simulink model "cp_aero_machineside"  (R2023b)
settings: Solver=VariableStepAuto  StartTime=0.0  StopTime=100  RelTol=1e-3
undefined symbols (not defined in the file): c_drt, C_p_opt, H_gen, H_WTR, k_drt, K_pitch, ki, kp, L_d, L_q, lambda_opt, omega_WTR_0, omega_WTR_min, omega_WTR_n, omega_WTR_sl0, pitch_max, pitch_min, poles, psi_pm, R_a, R_WTR, rate_max, rate_min, T_pitch, T_servo, v_w_n, wind_array_step
libraries: spsdq0toabcLib x1
settings Model: Creator=Martin Pedersen  LastModifiedBy=s183702

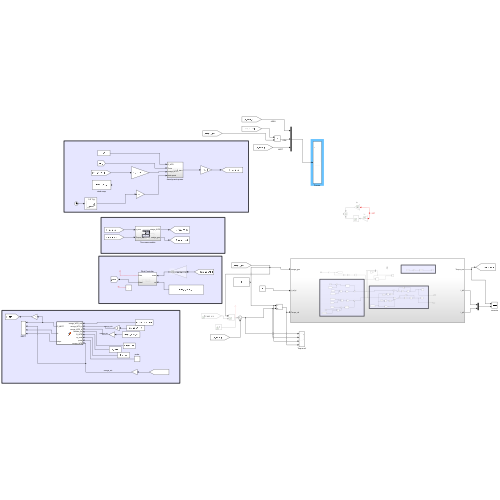
[thumbnail: Simulink's stored preview of the top-level diagram]
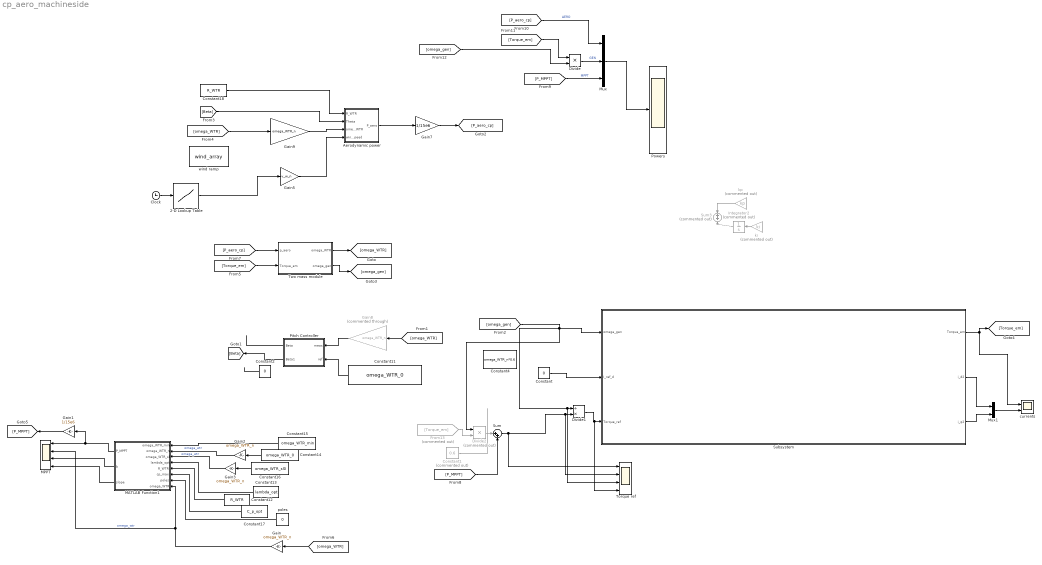
== system cp_aero_machineside ==
  2-D Lookup Table : Lookup_n-D  NumberOfTableDimensions=1  BreakpointsForDimension1=wind_array_step(1,:)  BreakpointsForDimension2=[1:3]  IndexSearchMethod=Linear search  Table=wind_array_step(2,:)  InterpMethod=Nearest  InternalRulePriority=Speed  RndMeth=Simplest
  Aerodynamic power : Subsystem
  Clock : Clock
  Constant : Constant  Value=0
  Constant1 : Constant  Commented=on  Value=0.6
  Constant11 : Constant  Value=omega_WTR_0
  Constant12 : Constant  Value=R_WTR
  Constant13 : Constant  Value=lambda_opt
  Constant14 : Constant  Value=omega_WTR_0
  Constant15 : Constant  Value=omega_WTR_min
  Constant16 : Constant  Value=omega_WTR_sl0
  Constant17 : Constant  Value=C_p_opt
  Constant18 : Constant  Value=R_WTR
  Constant2 : Constant  Value=0
  Constant4 : Constant  Value=omega_WTR_n*0.6
  Divide : Product  Inputs=**
  Divide1 : Product  Inputs=/*
  Divide2 : Product  Commented=on  Inputs=**
  From13 : From  Commented=on  GotoTag=Torque_em
  Gain{,2..3,9} (4 alike) : Gain  Gain=omega_WTR_n
  Gain1 : Gain  Gain=1/15e6
  Gain5 : Gain  Gain=v_w_n
  Gain7 : Gain  Gain=1/15e6
  Gain8 : Gain  Commented=through  Gain=omega_WTR_n
  Integrator2 : Integrator  Commented=on
  MATLAB Function1 : MATLAB Function  TreatAsAtomicUnit=on
  MPPT : Scope  NumInputPorts=4
  Mux : Mux  Inputs=3
  Mux1 : Mux  Inputs=2
  Pitch Controller : Subsystem
  Powers : Scope
  Subsystem : Subsystem
  Sum : Sum  Inputs=|++
  Sum3 : Sum  Commented=on  Inputs=+|+
  Torque ref : Scope  NumInputPorts=4
  Two mass module : Subsystem
  currents : Scope  NumInputPorts=2
  ki : Gain  Commented=on  Gain=ki
  kp : Gain  Commented=on  Gain=kp
  poles : Constant  Value=0
  wind ramp : FromWorkspace  VariableName=wind_array
  wires:
  Gain7/1 -> [P_aero_cp]
  [omega_WTR] -> Gain9/1
  Constant18/1 -> Aerodynamic power/1(R_WTR)
  [Beta] -> Aerodynamic power/2(Theta)
  Gain9/1 -> Aerodynamic power/3(omega_WTR)
  Gain5/1 -> Aerodynamic power/4(wind speed)
  Aerodynamic power/1(P_aero) -> Gain7/1
  MATLAB Function1/3(slope) -> MPPT/4
  MATLAB Function1/2(b) -> MPPT/3
  MATLAB Function1/1(P_MPPT) -> Gain1/1, MPPT/1
  Constant16/1 -> Gain3/1
  Constant17/1 -> MATLAB Function1/6(cp_max)
  Constant13/1 -> MATLAB Function1/4(lambda_opt)
  poles/1 -> MATLAB Function1/7(poles)
  Gain/1 -> MATLAB Function1/8(omega_WTR), MPPT/2  "omega_wtr"
  Constant12/1 -> MATLAB Function1/5(R_WTR)
  Constant14/1 -> Gain2/1
  Constant15/1 -> MATLAB Function1/1(omega_WTR_min)
  Two mass module/1(omega_WTR) -> [omega_WTR]
  [omega_WTR] -> Gain8/1
  Gain8/1 -> Pitch Controller/1(meas)
  Constant11/1 -> Pitch Controller/2(ref)
  kp/1 -> Sum3/1
  ? -> ki/1, kp/1
  ki/1 -> Integrator2/1
  Integrator2/1 -> Sum3/2
  Two mass module/2(omega_gen) -> [omega_gen]
  Subsystem/1(Torque_em) -> [Torque_em], currents/1
  [Torque_em] -> Two mass module/2(Torque_em)
  [omega_WTR] -> Gain/1
  [P_aero_cp] -> Two mass module/1(p_aero)
  Constant/1 -> Subsystem/2(I_ref_d)
  [P_MPPT] -> Mux/3  "MPPT"
  [P_aero_cp] -> Mux/1  "AERO"
  Divide/1 -> Mux/2  "GEN"
  [Torque_em] -> Divide/1
  Gain1/1 -> [P_MPPT]
  Mux1/1 -> currents/2
  Subsystem/2(i_d2) -> Mux1/1
  Subsystem/3(i_q2) -> Mux1/2
  Mux/1 -> Powers/1
  Pitch Controller/1(Beta) -> ?
  2-D Lookup Table/1 -> Gain5/1
  [omega_gen] -> Divide/2
  Constant2/1 -> ?
  Divide1/1 -> Torque ref/4, Subsystem/3(Torque_ref)
  Divide2/1 -> ?
  [P_MPPT] -> Sum/2
  Sum/1 -> Torque ref/2, Divide1/2, Torque ref/1
  Constant1/1 -> Sum/1
  From13/1 -> Divide2/2
  Gain2/1 -> MATLAB Function1/2(omega_WTR_n)  "omega_wtr"
  Gain3/1 -> MATLAB Function1/3(omega_WTR_sl)  "omega_wtr"
  [omega_gen] -> Torque ref/3, Divide1/1, Divide2/1, Subsystem/1(omega_gen)
  Pitch Controller/2(Beta1) -> [Beta]
  Clock/1 -> 2-D Lookup Table/1

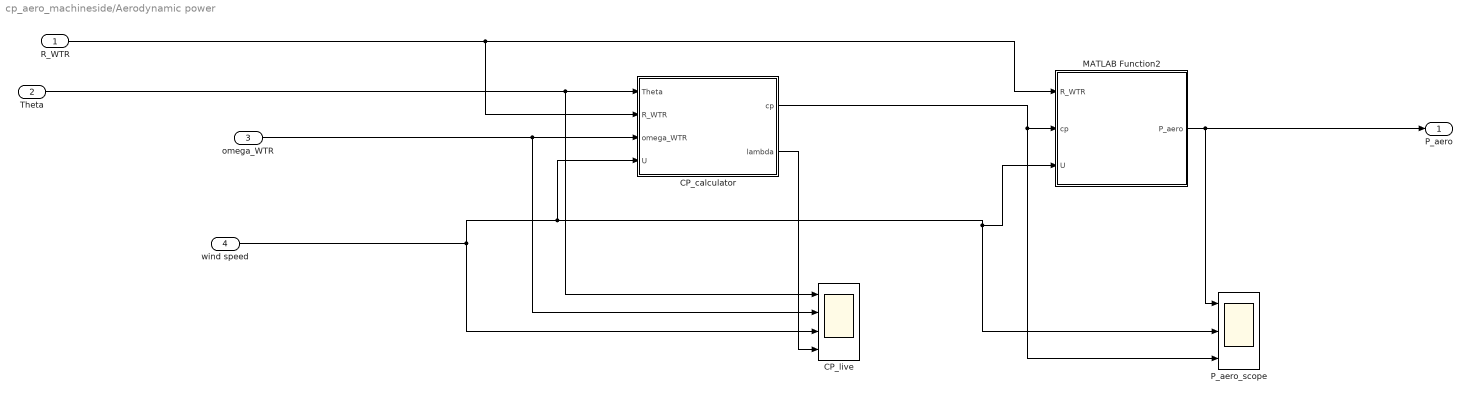
== system cp_aero_machineside/Aerodynamic power ==
  R_WTR : Inport
  Theta : Inport  Port=2
  omega_WTR : Inport  Port=3
  wind speed : Inport  Port=4
  CP_calculator : MATLAB Function  TreatAsAtomicUnit=on
  CP_live : Scope  NumInputPorts=4
  MATLAB Function2 : MATLAB Function  TreatAsAtomicUnit=on
  P_aero_scope : Scope  NumInputPorts=3
  P_aero : Outport
  wires:
  R_WTR/1 -> CP_calculator/2(R_WTR), MATLAB Function2/1(R_WTR)
  CP_calculator/1(cp) -> P_aero_scope/3, MATLAB Function2/2(cp)
  wind speed/1 -> P_aero_scope/2, MATLAB Function2/3(U), CP_calculator/4(U), CP_live/3
  Theta/1 -> CP_live/1, CP_calculator/1(Theta)
  omega_WTR/1 -> CP_calculator/3(omega_WTR), CP_live/2
  MATLAB Function2/1(P_aero) -> P_aero/1, P_aero_scope/1
  CP_calculator/2(lambda) -> CP_live/4

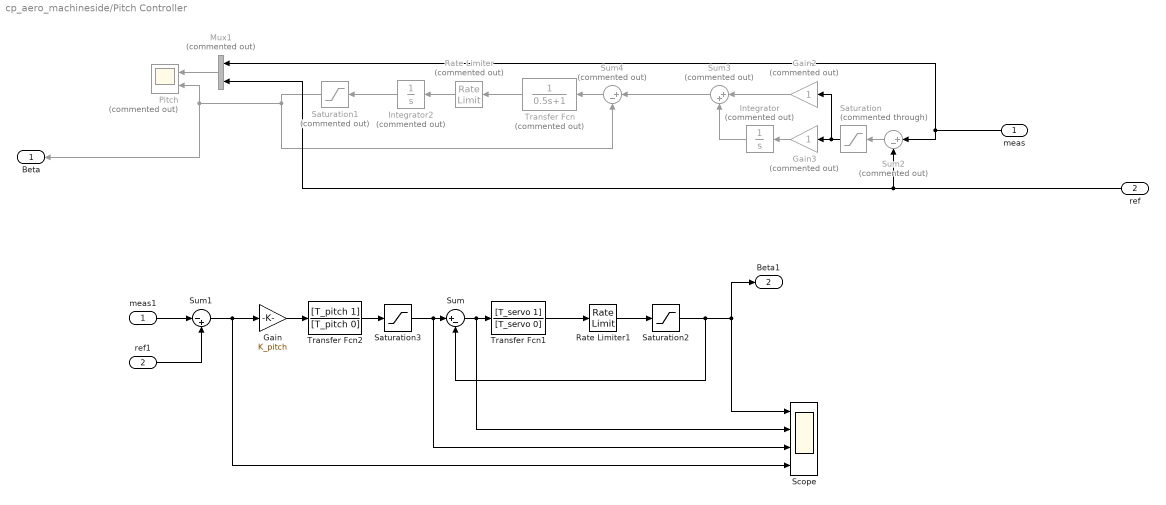
== system cp_aero_machineside/Pitch Controller ==
  meas : Inport
  ref : Inport  Port=2
  Gain : Gain  Gain=K_pitch
  Gain2 : Gain  Commented=on
  Gain3 : Gain  Commented=on
  Integrator : Integrator  Commented=on
  Integrator2 : Integrator  Commented=on
  Mux1 : Mux  Commented=on  Inputs=2
  Pitch : Scope  Commented=on  NumInputPorts=2
  Rate Limiter : RateLimiter  Commented=on  RisingSlewLimit=5  FallingSlewLimit=-5  SampleTimeMode=inherited
  Rate Limiter1 : RateLimiter  RisingSlewLimit=rate_max  FallingSlewLimit=rate_min  SampleTimeMode=inherited
  Saturation : Saturate  Commented=through  UpperLimit=inf  LowerLimit=0
  Saturation1 : Saturate  Commented=on  UpperLimit=90  LowerLimit=0
  Saturation2 : Saturate  UpperLimit=pitch_max  LowerLimit=pitch_min
  Saturation3 : Saturate  UpperLimit=pitch_max  LowerLimit=pitch_min
  Scope : Scope  NumInputPorts=4
  Sum : Sum  Inputs=|+-
  Sum1 : Sum  Inputs=|-+
  Sum2 : Sum  Commented=on  Inputs=|+-
  Sum3 : Sum  Commented=on  Inputs=|++
  Sum4 : Sum  Commented=on  Inputs=|+-
  Transfer Fcn : TransferFcn  Commented=on  Denominator=[0.5 1]
  Transfer Fcn1 : TransferFcn  Numerator=[T_servo 1]  Denominator=[T_servo 0]
  Transfer Fcn2 : TransferFcn  Numerator=[T_pitch 1]  Denominator=[T_pitch 0]
  meas1 : InportShadow
  ref1 : InportShadow  Port=2
  Beta : Outport
  Beta1 : Outport  Port=2
  wires:
  Transfer Fcn/1 -> Rate Limiter/1
  meas/1 -> Sum2/1, Mux1/1
  Mux1/1 -> Pitch/1
  Sum2/1 -> Saturation/1
  Sum3/1 -> Sum4/1
  Saturation/1 -> Gain2/1, Gain3/1
  Saturation1/1 -> Beta/1, Pitch/2, Sum4/2
  Gain3/1 -> Integrator/1
  Gain2/1 -> Sum3/1
  Sum4/1 -> Transfer Fcn/1
  Rate Limiter/1 -> Integrator2/1
  Integrator/1 -> Sum3/2
  ref/1 -> Mux1/2, Sum2/2
  Integrator2/1 -> Saturation1/1
  Rate Limiter1/1 -> Saturation2/1
  Gain/1 -> Transfer Fcn2/1
  Sum/1 -> Scope/2, Transfer Fcn1/1
  Transfer Fcn2/1 -> Saturation3/1
  Transfer Fcn1/1 -> Rate Limiter1/1
  Saturation2/1 -> Beta1/1, Scope/1, Sum/2
  Sum1/1 -> Gain/1, Scope/4
  meas1/1 -> Sum1/1
  ref1/1 -> Sum1/2
  Saturation3/1 -> Scope/3, Sum/1

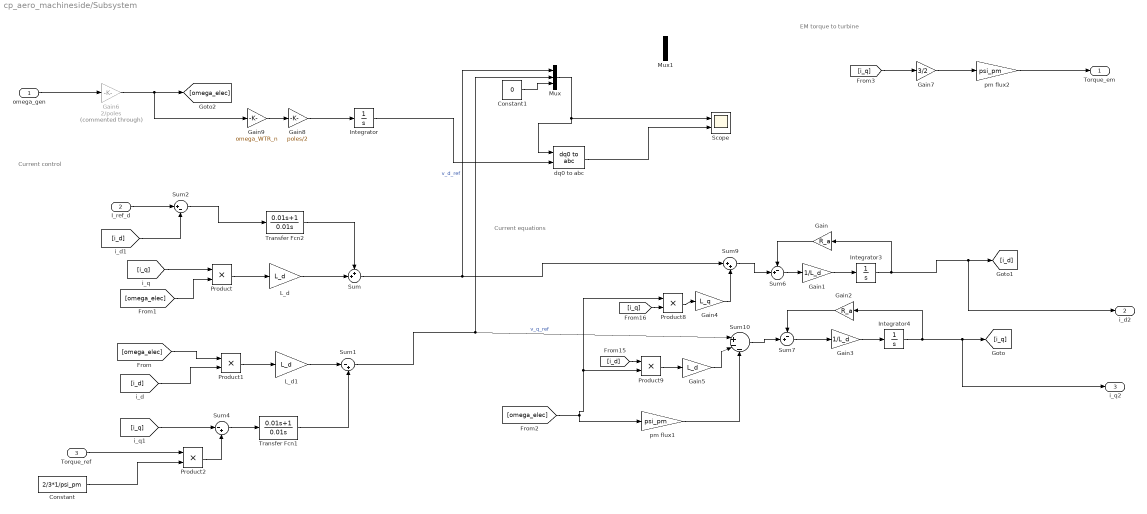
== system cp_aero_machineside/Subsystem ==
  note: EM torque to turbine
  note: Current control
  note: Current equations
  omega_gen : Inport
  I_ref_d : Inport  Port=2
  Torque_ref : Inport  Port=3
  Constant : Constant  Value=2/3*1/psi_pm
  Constant1 : Constant  Value=0
  Gain : Gain  Gain=R_a
  Gain1 : Gain  Gain=1/L_d
  Gain2 : Gain  Gain=R_a
  Gain3 : Gain  Gain=1/L_d
  Gain4 : Gain  Gain=L_q
  Gain5 : Gain  Gain=L_d
  Gain6 : Gain  Commented=through  Gain=2/poles
  Gain7 : Gain  Gain=3/2
  Gain8 : Gain  Gain=poles/2
  Gain9 : Gain  Gain=omega_WTR_n
  Integrator : Integrator
  Integrator3 : Integrator
  Integrator4 : Integrator  InitialCondition=2.3e4
  L_d : Gain  Gain=L_d
  L_d1 : Gain  Gain=L_d
  Mux : Mux  Inputs=3
  Mux1 : Mux  Inputs=3
  Product{,1..2,8..9} (5 alike) : Product
  Scope : Scope  NumInputPorts=2
  Sum : Sum  Inputs=++|
  Sum1 : Sum  Inputs=|-+
  Sum10 : Sum  Inputs=|+--
  Sum2 : Sum  Inputs=|+-
  Sum4 : Sum  Inputs=|-+
  Sum6 : Sum  Inputs=-+|
  Sum7 : Sum  Inputs=-+|
  Sum9 : Sum  Inputs=|++
  Transfer Fcn1 : TransferFcn  Numerator=[0.01 1]  Denominator=[0.01 0]
  Transfer Fcn2 : TransferFcn  Numerator=[0.01 1]  Denominator=[0.01 0]
  dq0 to abc : spsdq0toabcLib/dq0 to abc  Alignment=90 degrees behind phase A axis
  pm flux1 : Gain  Gain=psi_pm
  pm flux2 : Gain  Gain=psi_pm
  Torque_em : Outport
  i_d2 : Outport  Port=2
  i_q2 : Outport  Port=3
  wires:
  [i_q] -> Product/1
  [omega_elec] -> Product/2
  Product/1 -> L_d/1
  L_d/1 -> Sum/2
  [omega_elec] -> Product1/1
  [i_d] -> Product1/2
  Torque_ref/1 -> Product2/1
  Constant/1 -> Product2/2
  [i_d] -> Sum2/2
  I_ref_d/1 -> Sum2/1
  Sum2/1 -> Transfer Fcn2/1
  Transfer Fcn2/1 -> Sum/1
  Product2/1 -> Sum4/2
  [i_q] -> Sum4/1
  Sum1/1 -> Mux/2, Sum10/1  "v_q_ref"
  Sum/1 -> Mux/1, Sum9/1  "v_d_ref"
  Transfer Fcn1/1 -> Sum1/2
  Sum4/1 -> Transfer Fcn1/1
  Product8/1 -> Gain4/1
  [omega_elec] -> Product8/1, Product9/2, pm flux1/1
  pm flux1/1 -> Sum10/3
  [i_q] -> Product8/2
  Product9/1 -> Gain5/1
  Gain4/1 -> Sum9/2
  [i_d] -> Product9/1
  Gain5/1 -> Sum10/2
  Gain1/1 -> Integrator3/1
  Integrator3/1 -> Gain/1, i_d2/1, [i_d]
  Sum6/1 -> Gain1/1
  Sum9/1 -> Sum6/2
  Gain/1 -> Sum6/1
  Gain2/1 -> Sum7/1
  Sum7/1 -> Gain3/1
  Sum10/1 -> Sum7/2
  Gain3/1 -> Integrator4/1
  omega_gen/1 -> Gain6/1
  pm flux2/1 -> Torque_em/1
  Gain7/1 -> pm flux2/1
  [i_q] -> Gain7/1
  Integrator4/1 -> i_q2/1, [i_q], Gain2/1
  Gain6/1 -> Gain9/1, [omega_elec]
  L_d1/1 -> Sum1/1
  Product1/1 -> L_d1/1
  Constant1/1 -> Mux/3
  Mux/1 -> Scope/1, dq0 to abc/1
  Gain8/1 -> Integrator/1
  Gain9/1 -> Gain8/1
  Integrator/1 -> dq0 to abc/2
  dq0 to abc/1 -> Scope/2

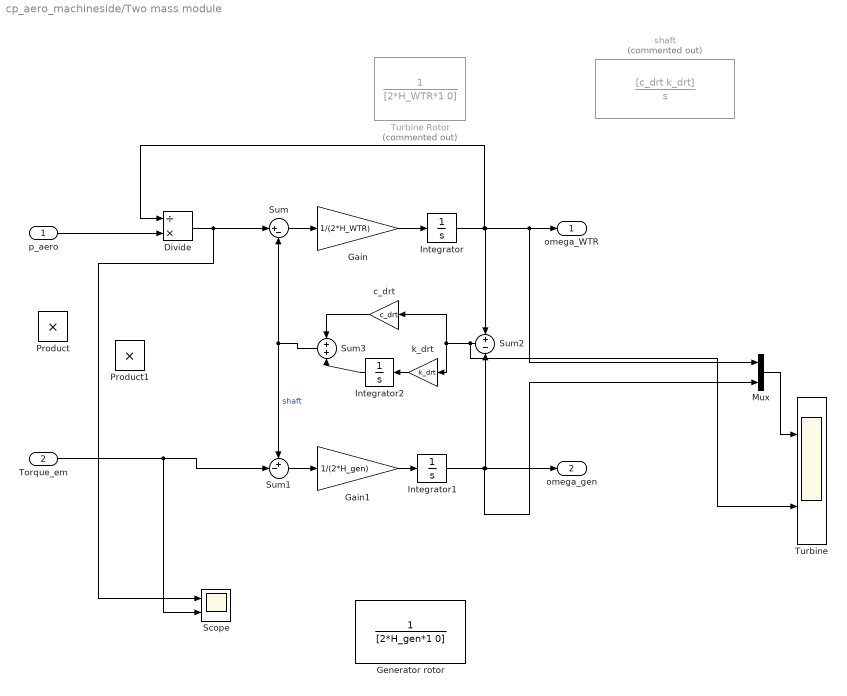
== system cp_aero_machineside/Two mass module ==
  p_aero : Inport
  Torque_em : Inport  Port=2
  Divide : Product  Inputs=/*
  Gain : Gain  Gain=1/(2*H_WTR)
  Gain1 : Gain  Gain=1/(2*H_gen)
  Generator rotor : TransferFcn  Denominator=[2*H_gen*1 0]
  Integrator : Integrator  InitialCondition=omega_WTR_0
  Integrator1 : Integrator  InitialCondition=omega_WTR_0
  Integrator2 : Integrator
  Mux : Mux  Inputs=2
  Product : Product
  Product1 : Product
  Scope : Scope  NumInputPorts=2
  Sum : Sum  Inputs=|+-
  Sum1 : Sum  Inputs=+-|
  Sum2 : Sum  Inputs=+|-
  Sum3 : Sum  Inputs=+|+
  Turbine : Scope  NumInputPorts=2
  Turbine Rotor : TransferFcn  Commented=on  Denominator=[2*H_WTR*1 0]
  c_drt : Gain  Gain=c_drt
  k_drt : Gain  Gain=k_drt
  shaft : TransferFcn  Commented=on  Numerator=[c_drt k_drt]  Denominator=[1 0]
  omega_WTR : Outport
  omega_gen : Outport  Port=2
  wires:
  Torque_em/1 -> Scope/2, Sum1/2
  Integrator1/1 -> omega_gen/1, Sum2/2, Mux/2
  Sum3/1 -> Sum1/1, Sum/2  "shaft"
  Integrator/1 -> Divide/1, Mux/1, omega_WTR/1, Sum2/1
  Sum/1 -> Gain/1
  p_aero/1 -> Divide/2
  Gain/1 -> Integrator/1
  Gain1/1 -> Integrator1/1
  Sum1/1 -> Gain1/1
  Integrator2/1 -> Sum3/2
  c_drt/1 -> Sum3/1
  Sum2/1 -> Turbine/2, k_drt/1, c_drt/1
  k_drt/1 -> Integrator2/1
  Mux/1 -> Turbine/1
  Divide/1 -> Scope/1, Sum/1

== matlab function cp_aero_machineside/MATLAB Function1 ==
  data: omega_WTR_min input; P_MPPT output; omega_WTR_n input; omega_WTR_sl input; lambda_opt input; R_WTR input; cp_max input; poles input; omega_WTR input; b output; slope output
function [P_MPPT,b,slope] = fcn(omega_WTR_min,omega_WTR_n,omega_WTR_sl,lambda_opt,R_WTR,cp_max,poles,omega_WTR)

rho = 1.2225;
P_mppt_sl = 0.5*pi*rho*R_WTR^5*cp_max/lambda_opt^3*omega_WTR_sl^3; %
P_mppt_max = 0.5*pi*rho*R_WTR^5*cp_max/lambda_opt^3*omega_WTR_n^3;
slope = (P_mppt_max-P_mppt_sl)/(omega_WTR_n-omega_WTR_sl);
b = P_mppt_max-slope*omega_WTR_n;

if omega_WTR < omega_WTR_min
    y = 0;
elseif omega_WTR < omega_WTR_sl
    y = 0.5*pi*rho*R_WTR^5*cp_max/lambda_opt^3*omega_WTR^3;
elseif omega_WTR < omega_WTR_n
    y = slope*omega_WTR+b;
else
    y = 0.5*pi*rho*R_WTR^5*cp_max/lambda_opt^3*omega_WTR_n^3;

end

P_MPPT = y ;

== matlab function cp_aero_machineside/Aerodynamic power/MATLAB Function2 ==
  data: R_WTR input; cp input; P_aero output; U input
function P_aero = fcn(R_WTR,cp,U)

rho = 1.225;
P_aero = 0.5*pi*rho*R_WTR^2*cp*U^3;

== matlab function cp_aero_machineside/Aerodynamic power/CP_calculator ==
  data: Theta input; R_WTR input; omega_WTR input; cp output; U input; lambda output
function  [cp, lambda] = fcn(Theta,R_WTR,omega_WTR,U) 
    
    lambda = omega_WTR*R_WTR/U;

    c = [0.645 116 0.4 5 21 0.00912 0.08 0.035 0.001];
    a = (-c(4)-c(3)*(2.5+Theta)+c(2)*1/(lambda+c(7)*(2.5+Theta))-c(8)/(lambda+(2.5+Theta)^3));
    exponent = c(5)*1/(lambda+c(7)*(2.5+Theta))-c(8)/(lambda+(2.5+Theta)^3);
    x = c(1)*(c(6)*lambda+a/exp(exponent))+c(9)*lambda;

cp = x;
